simulink model "SF5_4_1_jc0742"  (R2016b)
settings: Solver=VariableStepAuto  StartTime=0.0  StopTime=10.0  RelTol=1e-3  EnableMultiTasking=on
settings Model: Creator=amyyang  LastModifiedBy=amyyang
settings DataIOCC: LimitDataPoints=on
settings OptimizationCC: LifeSpan=inf
settings DebuggingCC: AllowSymbolicDim=off  SFUnexpectedBacktrackingDiag=warning  SFNoUnconditionalDefaultTransitionDiag=warning  SFExecutionAtInitializationDiag=none
settings ModelReferenceCC: PropagateSignalLabelsOutOfModel=off
settings GRTTargetCC: TargetLangStandard=C89/C90 (ANSI)
settings ConfigComp: CovMetricSettings=dw  CovHtmlReporting=on  CovSaveCumulativeToWorkspaceVar=on  CovSaveSingleToWorkspaceVar=on  CovExternalEMLEnable=off

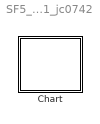
== system SF5_4_1_jc0742 ==
  Chart : Stateflow chart  TreatAsAtomicUnit=on

== stateflow chart SF5_4_1_jc0742/Chart ==
  state A
  state B
  state B1
  state A1
  state B2
  state A2
  state Incorrect1
  state B3
  A -> B : % 多个条件尽量写在一行
      | [ condition1 && condition2 && condition3]
  B -> A : [ ( condition1 && condition2) || condition3]
  A1 -> B1 : % 若需要分行，操作符的位置都统一写在条件后面或者前面
      | [ condition1 &&...
      |   condition2 &&...
      |   condition3]
  B1 -> A1 : [ ( condition1 && condition2) ||...
      |     condition3]
  B2 -> A2 : % 使用了不同类型的运算符，要使用括号把优先级显式表示出来
      | [  (condition1 && condition2) ||condition3]
  Incorrect1 -> B3 : % 不要把超过四个运算符写在同一行
      | [ condition1 && condition2 && condition3 && condition4]
